simulink subsystem "Joystick_Input_To_Swerve_Drive_sub"  (R2023b)
settings: Solver=VariableStepAuto  StartTime=0.0  StopTime=10.0  RelTol=1e-3
undefined symbols (not defined in the file): Boost_Trigger_High_Speed, Boost_Trigger_Low_Speed, Steering_Abs_Deadband_Range, Steering_Mod_Drv_in, Steering_Mod_Drv_out, Steering_Mod_Str_Rel_in, Steering_Mod_Str_Rel_out, Steering_Relative_Gain, Steering_Twist_Gain, Translation_Twist_Gain
libraries: simulink x12, hdlsllib x5, Controls_Components_lib x1
settings Model: Creator=ander  LastModifiedBy=ander

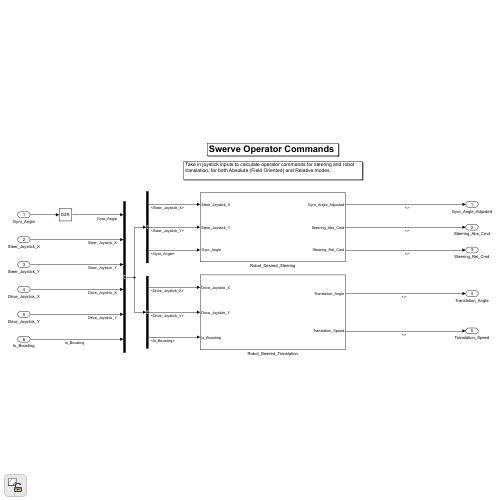
[thumbnail: Simulink's stored preview of the top-level diagram]
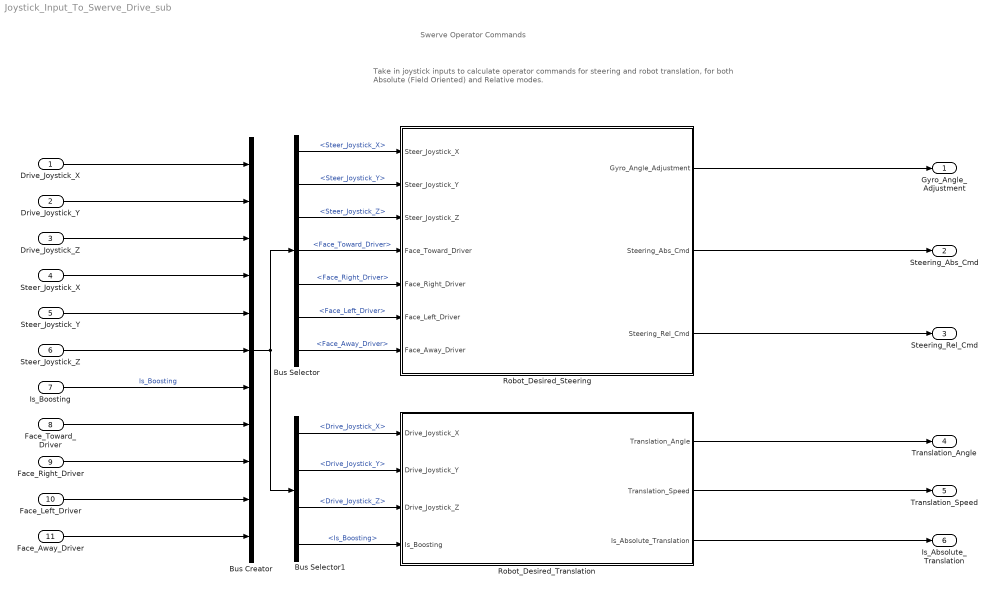
== system Joystick_Input_To_Swerve_Drive_sub ==
  note: Take in joystick inputs to calculate operator commands for steering and robot translation, for both Absolute (Field Oriented) and Relative modes.
  note: Swerve Operator Commands
  Drive_Joystick_X : Inport
  Drive_Joystick_Y : Inport  Port=2
  Drive_Joystick_Z : Inport  Port=3
  Steer_Joystick_X : Inport  Port=4
  Steer_Joystick_Y : Inport  Port=5
  Steer_Joystick_Z : Inport  Port=6
  Is_Boosting : Inport  Port=7
  Face_Toward_Driver : Inport  Port=8
  Face_Right_Driver : Inport  Port=9
  Face_Left_Driver : Inport  Port=10
  Face_Away_Driver : Inport  Port=11
  Bus Creator : BusCreator  Inputs=11
  Bus Selector : BusSelector  OutputSignals=Steer_Joystick_X,Steer_Joystick_Y,Steer_Joystick_Z,Face_Toward_Driver,Face_Right_Driver,Face_Left_Driver,Face_Away_Driver
  Bus Selector1 : BusSelector  OutputSignals=Drive_Joystick_X,Drive_Joystick_Y,Drive_Joystick_Z,Is_Boosting
  Robot_Desired_Steering : Subsystem
  Robot_Desired_Translation : Subsystem
  Gyro_Angle_Adjustment : Outport
  Steering_Abs_Cmd : Outport  Port=2
  Steering_Rel_Cmd : Outport  Port=3
  Translation_Angle : Outport  Port=4
  Translation_Speed : Outport  Port=5
  Is_Absolute_Translation : Outport  Port=6
  wires:
  Bus Selector/7 -> Robot_Desired_Steering/7(Face_Away_Driver)  "<Face_Away_Driver>"
  Bus Selector/6 -> Robot_Desired_Steering/6(Face_Left_Driver)  "<Face_Left_Driver>"
  Bus Selector/5 -> Robot_Desired_Steering/5(Face_Right_Driver)  "<Face_Right_Driver>"
  Bus Selector/3 -> Robot_Desired_Steering/3(Steer_Joystick_Z)  "<Steer_Joystick_Z>"
  Bus Selector/4 -> Robot_Desired_Steering/4(Face_Toward_Driver)  "<Face_Toward_Driver>"
  Is_Boosting/1 -> Bus Creator/7  "Is_Boosting"
  Face_Away_Driver/1 -> Bus Creator/11
  Face_Left_Driver/1 -> Bus Creator/10
  Face_Right_Driver/1 -> Bus Creator/9
  Face_Toward_Driver/1 -> Bus Creator/8
  Steer_Joystick_Z/1 -> Bus Creator/6
  Steer_Joystick_X/1 -> Bus Creator/4
  Drive_Joystick_Y/1 -> Bus Creator/2
  Steer_Joystick_Y/1 -> Bus Creator/5
  Drive_Joystick_Z/1 -> Bus Creator/3
  Drive_Joystick_X/1 -> Bus Creator/1
  Bus Selector1/1 -> Robot_Desired_Translation/1(Drive_Joystick_X)  "<Drive_Joystick_X>"
  Bus Selector1/2 -> Robot_Desired_Translation/2(Drive_Joystick_Y)  "<Drive_Joystick_Y>"
  Bus Creator/1 -> Bus Selector1/1, Bus Selector/1
  Robot_Desired_Translation/2(Translation_Speed) -> Translation_Speed/1
  Robot_Desired_Translation/1(Translation_Angle) -> Translation_Angle/1
  Bus Selector/1 -> Robot_Desired_Steering/1(Steer_Joystick_X)  "<Steer_Joystick_X>"
  Bus Selector/2 -> Robot_Desired_Steering/2(Steer_Joystick_Y)  "<Steer_Joystick_Y>"
  Robot_Desired_Steering/1(Gyro_Angle_Adjustment) -> Gyro_Angle_Adjustment/1
  Robot_Desired_Steering/2(Steering_Abs_Cmd) -> Steering_Abs_Cmd/1
  Robot_Desired_Steering/3(Steering_Rel_Cmd) -> Steering_Rel_Cmd/1
  Bus Selector1/4 -> Robot_Desired_Translation/4(Is_Boosting)  "<Is_Boosting>"
  Bus Selector1/3 -> Robot_Desired_Translation/3(Drive_Joystick_Z)  "<Drive_Joystick_Z>"
  Robot_Desired_Translation/3(Is_Absolute_Translation) -> Is_Absolute_Translation/1

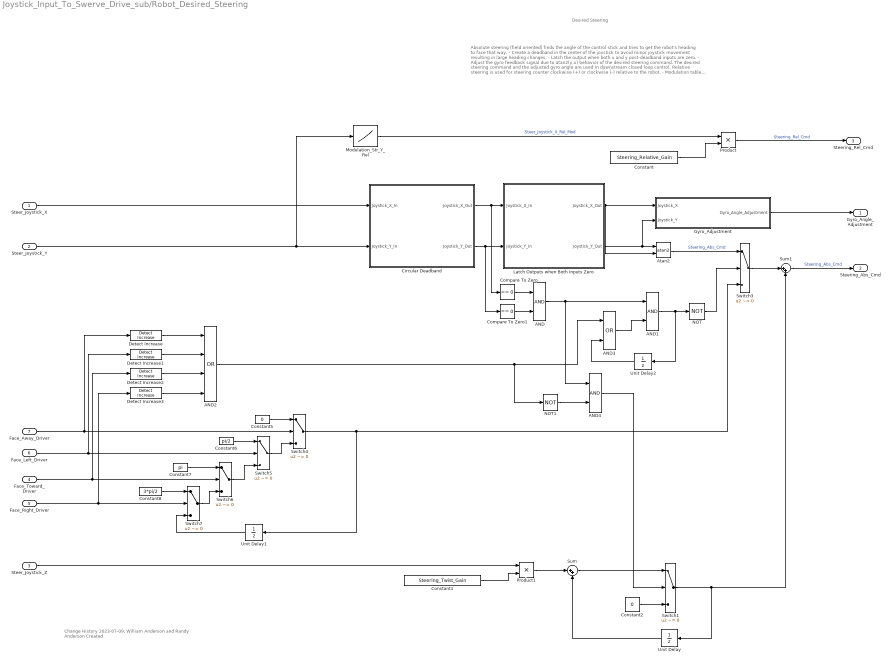
== system Joystick_Input_To_Swerve_Drive_sub/Robot_Desired_Steering ==
  note: Absolute steering (field oriented) finds the angle of the control stick and tries to get the robot's heading to face that way.
      | - Create a deadband in the center of the joystick to avoid minor joystick movement resulting in large heading changes.
      | - Latch the output when both x and y post-deadband inputs are zero.
      | - Adjust the gyro feedback signal due to atan2(y,x) behavior of the desired steering command. The desired steering command and the adjusted gyro angle are used in downstream closed loop control.
      |
      | Relative steering is used for steering counter clockwise (+) or clockwise (-) relative to the robot.
      | - Modulation table for joystick input. Only one axis of the steering joystck is used.
      | - The gain block adjusts how fast the robot will rotate.
  note: Desired Steering
  note: Change History
      | 2023-07-09, William Anderson and Randy Anderson
      | Created
  Steer_Joystick_X : Inport
  Steer_Joystick_Y : Inport  Port=2
  Steer_Joystick_Z : Inport  Port=3
  Face_Toward_Driver : Inport  Port=4
  Face_Right_Driver : Inport  Port=5
  Face_Left_Driver : Inport  Port=6
  Face_Away_Driver : Inport  Port=7
  AND : Logic  AllPortsSameDT=off  OutDataTypeStr=boolean
  AND1 : Logic  AllPortsSameDT=off  OutDataTypeStr=boolean
  AND2 : Logic  Operator=OR  Inputs=4  AllPortsSameDT=off  OutDataTypeStr=boolean
  AND3 : Logic  Operator=OR  AllPortsSameDT=off  OutDataTypeStr=boolean
  AND4 : Logic  AllPortsSameDT=off  OutDataTypeStr=boolean
  Atan2 : Trigonometry  Operator=atan2
  Circular Deadband : Subsystem
  Compare To Zero : simulink/Logic and Bit Operations/Compare To Zero  relop===  OutDataTypeStr=boolean
  Compare To Zero1 : simulink/Logic and Bit Operations/Compare To Zero  relop===  OutDataTypeStr=boolean
  Constant : Constant  Value=Steering_Relative_Gain
  Constant1 : Constant  Value=Steering_Twist_Gain
  Constant2 : Constant  Value=0
  Constant5 : Constant  Value=0
  Constant6 : Constant  Value=pi/2
  Constant7 : Constant  Value=pi
  Constant8 : Constant  Value=3*pi/2
  Detect Increase{,1..3} (4 alike) : simulink/Logic and Bit Operations/Detect Increase  vinit=0.0  OutDataTypeStr=boolean
  Gyro_Adjustment : Subsystem
  Latch Outputs when Both Inputs Zero : Subsystem
  Modulation_Str_Y_Rel : Lookup_n-D  NumberOfTableDimensions=1  BreakpointsForDimension1=Steering_Mod_Str_Rel_in  Table=Steering_Mod_Str_Rel_out  ExtrapMethod=Clip  InternalRulePriority=Speed  RndMeth=Simplest
  NOT : Logic  Operator=NOT  AllPortsSameDT=off  OutDataTypeStr=boolean
  NOT1 : Logic  Operator=NOT  AllPortsSameDT=off  OutDataTypeStr=boolean
  Product : Product
  Product1 : Product
  Sum : Sum  Inputs=|++
  Sum1 : Sum  Inputs=|++
  Switch{1,3..7} (6 alike) : Switch  Criteria=u2 ~= 0  SaturateOnIntegerOverflow=off  InputSameDT=off
  Unit Delay : UnitDelay  SampleTime=-1  HasFrameUpgradeWarning=on
  Unit Delay1 : UnitDelay  SampleTime=-1  HasFrameUpgradeWarning=on
  Unit Delay2 : UnitDelay  SampleTime=-1  HasFrameUpgradeWarning=on
  Gyro_Angle_Adjustment : Outport
  Steering_Abs_Cmd : Outport  Port=2
  Steering_Rel_Cmd : Outport  Port=3
  wires:
  NOT1/1 -> AND4/2
  AND4/1 -> Switch1/2
  Unit Delay2/1 -> AND3/2
  AND3/1 -> AND1/2
  AND1/1 -> NOT/1, Unit Delay2/1
  AND2/1 -> AND3/1, NOT1/1
  Detect Increase3/1 -> AND2/4
  Detect Increase2/1 -> AND2/3
  Detect Increase1/1 -> AND2/2
  Detect Increase/1 -> AND2/1
  Switch3/1 -> Sum1/1
  Atan2/1 -> Switch3/1  "Steering_Abs_Cmd"
  NOT/1 -> Switch3/2
  Unit Delay1/1 -> Switch7/3
  Switch4/1 -> Switch3/3, Unit Delay1/1
  Unit Delay/1 -> Sum/2
  Sum/1 -> Switch1/1
  Latch Outputs when Both Inputs Zero/1(Joystick_X_Out) -> Gyro_Adjustment/1(Joystick_X), Atan2/2
  Circular Deadband/1(Joystick_X_Out) -> Compare To Zero/1, Latch Outputs when Both Inputs Zero/1(Joystick_X_In)
  Circular Deadband/2(Joystick_Y_Out) -> Latch Outputs when Both Inputs Zero/2(Joystick_Y_In), Compare To Zero1/1
  Steer_Joystick_Y/1 -> Circular Deadband/2(Joystick_Y_In), Modulation_Str_Y_Rel/1
  Latch Outputs when Both Inputs Zero/2(Joystick_Y_Out) -> Atan2/1, Gyro_Adjustment/2(Joystick_Y)
  Gyro_Adjustment/1(Gyro_Angle_Adjustment) -> Gyro_Angle_Adjustment/1
  Sum1/1 -> Steering_Abs_Cmd/1  "Steering_Abs_Cmd"
  Constant/1 -> Product/2
  Product/1 -> Steering_Rel_Cmd/1  "Steering_Rel_Cmd"
  Steer_Joystick_X/1 -> Circular Deadband/1(Joystick_X_In)
  Modulation_Str_Y_Rel/1 -> Product/1  "Steer_Joystick_X_Rel_Mod"
  Steer_Joystick_Z/1 -> Product1/1
  Compare To Zero/1 -> AND/1
  Compare To Zero1/1 -> AND/2
  AND/1 -> AND1/1, AND4/1
  Constant2/1 -> Switch1/3
  Switch1/1 -> Unit Delay/1, Sum1/2
  Product1/1 -> Sum/1
  Constant1/1 -> Product1/2
  Constant5/1 -> Switch4/1
  Constant7/1 -> Switch6/1
  Switch6/1 -> Switch5/3
  Constant6/1 -> Switch5/1
  Constant8/1 -> Switch7/1
  Switch5/1 -> Switch4/3
  Switch7/1 -> Switch6/3
  Face_Away_Driver/1 -> Switch4/2, Detect Increase/1
  Face_Left_Driver/1 -> Switch5/2, Detect Increase1/1
  Face_Toward_Driver/1 -> Switch6/2, Detect Increase2/1
  Face_Right_Driver/1 -> Switch7/2, Detect Increase3/1

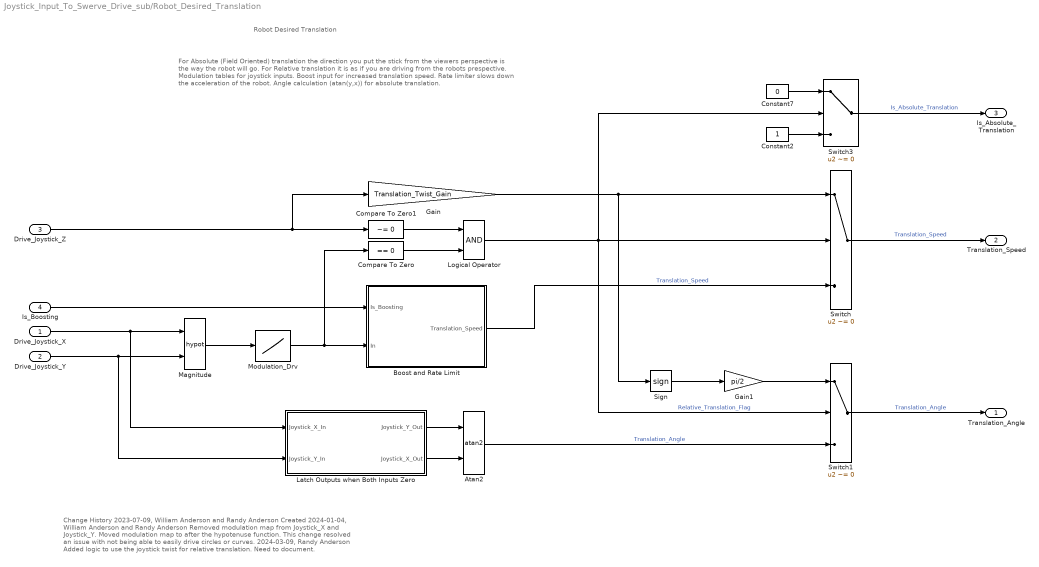
== system Joystick_Input_To_Swerve_Drive_sub/Robot_Desired_Translation ==
  note: Robot Desired Translation
  note: For Absolute (Field Oriented) translation the direction you put the stick from the viewers perspective is the way the robot will go.
      |
      | For Relative translation it is as if you are driving from the robots prespective.
      |
      | Modulation tables for joystick inputs.
      | Boost input for increased translation speed.
      | Rate limiter slows down the acceleration of the robot.
      | Angle calculation (atan(y,x)) for absolute translation.
  note: Change History
      | 2023-07-09, William Anderson and Randy Anderson
      | Created
      | 2024-01-04, William Anderson and Randy Anderson
      | Removed modulation map from Joystick_X and Joystick_Y.
      | Moved modulation map to after the hypotenuse function.
      | This change resolved an issue with not being able to easily drive circles or curves.
      | 2024-03-09, Randy Anderson
      | Added logic to use the joystick twist for relative translation. Need to document.
  Drive_Joystick_X : Inport
  Drive_Joystick_Y : Inport  Port=2
  Drive_Joystick_Z : Inport  Port=3
  Is_Boosting : Inport  Port=4
  Atan2 : Trigonometry  Operator=atan2
  Boost and Rate Limit : Subsystem
  Compare To Zero : simulink/Logic and Bit Operations/Compare To Zero  relop===  OutDataTypeStr=boolean
  Compare To Zero1 : simulink/Logic and Bit Operations/Compare To Zero  relop=~=  OutDataTypeStr=boolean
  Constant2 : Constant  OutDataTypeStr=Inherit: Inherit via back propagation
  Constant7 : Constant  Value=0  OutDataTypeStr=Inherit: Inherit via back propagation
  Gain : Gain  Gain=Translation_Twist_Gain
  Gain1 : Gain  Gain=pi/2
  Latch Outputs when Both Inputs Zero : Subsystem
  Logical Operator : Logic  AllPortsSameDT=off  OutDataTypeStr=boolean
  Magnitude : Math  Operator=hypot
  Modulation_Drv : Lookup_n-D  NumberOfTableDimensions=1  BreakpointsForDimension1=Steering_Mod_Drv_in  Table=Steering_Mod_Drv_out  ExtrapMethod=Clip  InternalRulePriority=Speed  RndMeth=Simplest
  Sign : Signum
  Switch : Switch  Criteria=u2 ~= 0  SaturateOnIntegerOverflow=off  InputSameDT=off
  Switch1 : Switch  Criteria=u2 ~= 0  SaturateOnIntegerOverflow=off  InputSameDT=off
  Switch3 : Switch  Criteria=u2 ~= 0  SaturateOnIntegerOverflow=off  InputSameDT=off
  Translation_Angle : Outport
  Translation_Speed : Outport  Port=2
  Is_Absolute_Translation : Outport  Port=3
  wires:
  Gain1/1 -> Switch1/1
  Sign/1 -> Gain1/1
  Switch3/1 -> Is_Absolute_Translation/1  "Is_Absolute_Translation"
  Constant7/1 -> Switch3/1
  Constant2/1 -> Switch3/3
  Atan2/1 -> Switch1/3  "Translation_Angle"
  Gain/1 -> Switch/1, Sign/1
  Compare To Zero/1 -> Logical Operator/2
  Compare To Zero1/1 -> Logical Operator/1
  Boost and Rate Limit/1(Translation_Speed) -> Switch/3  "Translation_Speed"
  Logical Operator/1 -> Switch3/2, Switch1/2, Switch/2  "Relative_Translation_Flag"
  Drive_Joystick_Z/1 -> Compare To Zero1/1, Gain/1
  Latch Outputs when Both Inputs Zero/1(Joystick_Y_Out) -> Atan2/1
  Latch Outputs when Both Inputs Zero/2(Joystick_X_Out) -> Atan2/2
  Is_Boosting/1 -> Boost and Rate Limit/1(Is_Boosting)
  Switch/1 -> Translation_Speed/1  "Translation_Speed"
  Switch1/1 -> Translation_Angle/1  "Translation_Angle"
  Magnitude/1 -> Modulation_Drv/1
  Drive_Joystick_X/1 -> Magnitude/1, Latch Outputs when Both Inputs Zero/1(Joystick_X_In)
  Drive_Joystick_Y/1 -> Magnitude/2, Latch Outputs when Both Inputs Zero/2(Joystick_Y_In)
  Modulation_Drv/1 -> Compare To Zero/1, Boost and Rate Limit/2(In)

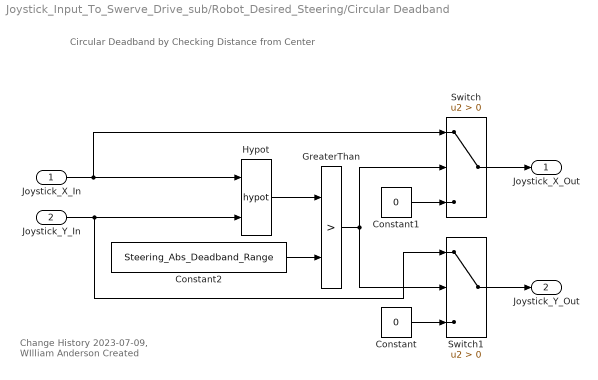
== system Joystick_Input_To_Swerve_Drive_sub/Robot_Desired_Steering/Circular Deadband ==
  note: Circular Deadband by Checking Distance from Center
  note: Change History
      | 2023-07-09, WIlliam Anderson
      | Created
  Joystick_X_In : Inport
  Joystick_Y_In : Inport  Port=2
  Constant : Constant  Value=0
  Constant1 : Constant  Value=0
  Constant2 : Constant  Value=Steering_Abs_Deadband_Range
  GreaterThan : RelationalOperator  Operator=>  OutDataTypeStr=boolean  RndMeth=Simplest  InputSameDT=off
  Hypot : Math  Operator=hypot
  Switch : Switch  Criteria=u2 > Threshold  SaturateOnIntegerOverflow=off  InputSameDT=off
  Switch1 : Switch  Criteria=u2 > Threshold  SaturateOnIntegerOverflow=off  InputSameDT=off
  Joystick_X_Out : Outport
  Joystick_Y_Out : Outport  Port=2
  wires:
  GreaterThan/1 -> Switch1/2, Switch/2
  Constant2/1 -> GreaterThan/2
  Hypot/1 -> GreaterThan/1
  Joystick_Y_In/1 -> Hypot/2, Switch1/1
  Joystick_X_In/1 -> Switch/1, Hypot/1
  Constant1/1 -> Switch/3
  Constant/1 -> Switch1/3
  Switch/1 -> Joystick_X_Out/1
  Switch1/1 -> Joystick_Y_Out/1

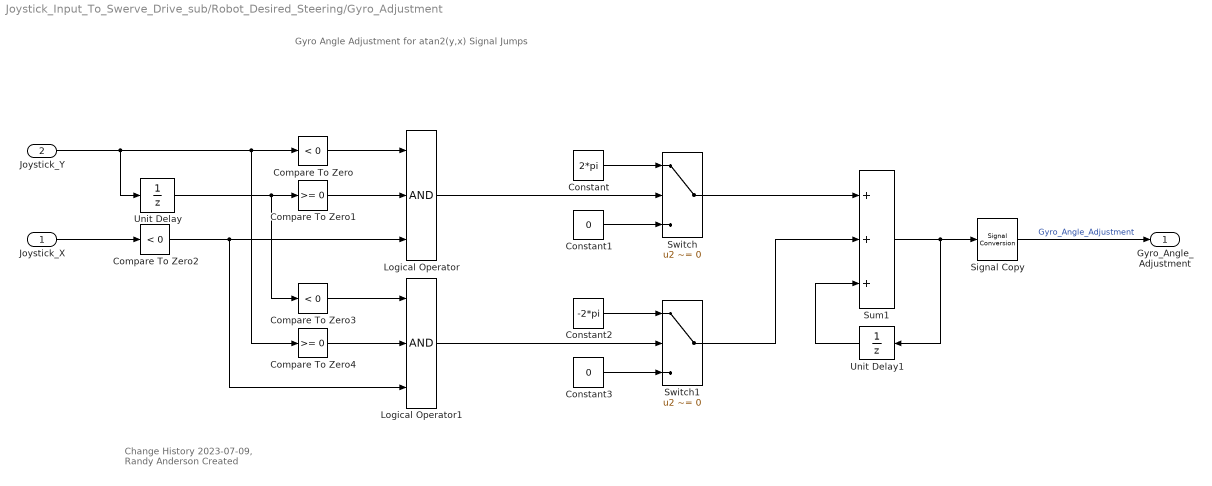
== system Joystick_Input_To_Swerve_Drive_sub/Robot_Desired_Steering/Gyro_Adjustment ==
  note: Gyro Angle Adjustment for atan2(y,x) Signal Jumps
  note: Change History
      | 2023-07-09, Randy Anderson
      | Created
  Joystick_X : Inport
  Joystick_Y : Inport  Port=2
  Compare To Zero : hdlsllib/Logic and Bit Operations/Compare To Zero  relop=<  OutDataTypeStr=boolean
  Compare To Zero1 : hdlsllib/Logic and Bit Operations/Compare To Zero  relop=>=  OutDataTypeStr=boolean
  Compare To Zero2 : hdlsllib/Logic and Bit Operations/Compare To Zero  relop=<  OutDataTypeStr=boolean
  Compare To Zero3 : hdlsllib/Logic and Bit Operations/Compare To Zero  relop=<  OutDataTypeStr=boolean
  Compare To Zero4 : hdlsllib/Logic and Bit Operations/Compare To Zero  relop=>=  OutDataTypeStr=boolean
  Constant : Constant  Value=2*pi
  Constant1 : Constant  Value=0
  Constant2 : Constant  Value=-2*pi
  Constant3 : Constant  Value=0
  Logical Operator : Logic  Inputs=3  AllPortsSameDT=off  OutDataTypeStr=boolean
  Logical Operator1 : Logic  Inputs=3  AllPortsSameDT=off  OutDataTypeStr=boolean
  Signal Copy : SignalConversion  OverrideOpt=off
  Sum1 : Sum  Inputs=3
  Switch : Switch  Criteria=u2 ~= 0  SaturateOnIntegerOverflow=off  InputSameDT=off
  Switch1 : Switch  Criteria=u2 ~= 0  SaturateOnIntegerOverflow=off  InputSameDT=off
  Unit Delay : UnitDelay  SampleTime=-1  HasFrameUpgradeWarning=on
  Unit Delay1 : UnitDelay  SampleTime=-1  HasFrameUpgradeWarning=on
  Gyro_Angle_Adjustment : Outport
  wires:
  Joystick_Y/1 -> Compare To Zero4/1, Compare To Zero/1, Unit Delay/1
  Unit Delay/1 -> Compare To Zero3/1, Compare To Zero1/1
  Compare To Zero/1 -> Logical Operator/1
  Compare To Zero1/1 -> Logical Operator/2
  Constant/1 -> Switch/1
  Constant1/1 -> Switch/3
  Logical Operator/1 -> Switch/2
  Sum1/1 -> Unit Delay1/1, Signal Copy/1
  Switch/1 -> Sum1/1
  Unit Delay1/1 -> Sum1/3
  Joystick_X/1 -> Compare To Zero2/1
  Compare To Zero2/1 -> Logical Operator1/3, Logical Operator/3
  Compare To Zero3/1 -> Logical Operator1/1
  Compare To Zero4/1 -> Logical Operator1/2
  Logical Operator1/1 -> Switch1/2
  Constant3/1 -> Switch1/3
  Constant2/1 -> Switch1/1
  Switch1/1 -> Sum1/2
  Signal Copy/1 -> Gyro_Angle_Adjustment/1  "Gyro_Angle_Adjustment"

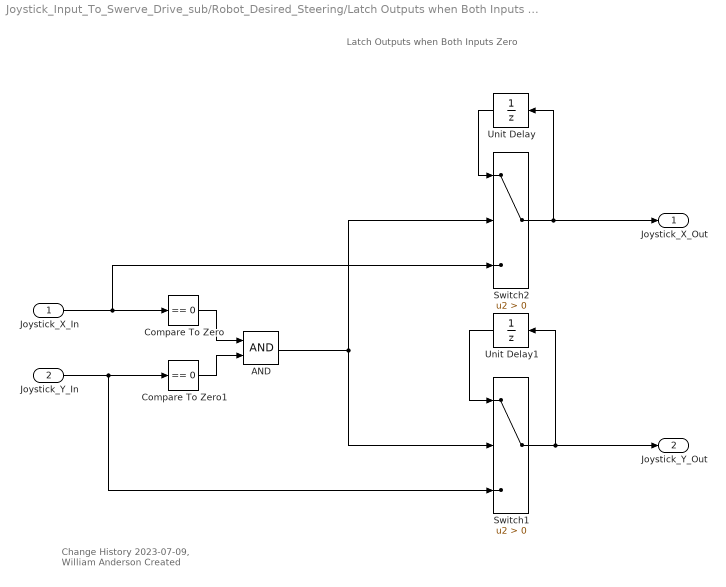
== system Joystick_Input_To_Swerve_Drive_sub/Robot_Desired_Steering/Latch Outputs when Both Inputs Zero ==
  note: Latch Outputs when Both Inputs Zero
  note: Change History
      | 2023-07-09, William Anderson
      | Created
  Joystick_X_In : Inport
  Joystick_Y_In : Inport  Port=2
  AND : Logic  AllPortsSameDT=off  OutDataTypeStr=boolean
  Compare To Zero : simulink/Logic and Bit Operations/Compare To Zero  relop===  OutDataTypeStr=boolean
  Compare To Zero1 : simulink/Logic and Bit Operations/Compare To Zero  relop===  OutDataTypeStr=boolean
  Switch1 : Switch  Criteria=u2 > Threshold  SaturateOnIntegerOverflow=off  InputSameDT=off
  Switch2 : Switch  Criteria=u2 > Threshold  SaturateOnIntegerOverflow=off  InputSameDT=off
  Unit Delay : UnitDelay  SampleTime=-1  HasFrameUpgradeWarning=on
  Unit Delay1 : UnitDelay  SampleTime=-1  HasFrameUpgradeWarning=on
  Joystick_X_Out : Outport
  Joystick_Y_Out : Outport  Port=2
  wires:
  Unit Delay1/1 -> Switch1/1
  Unit Delay/1 -> Switch2/1
  AND/1 -> Switch2/2, Switch1/2
  Compare To Zero/1 -> AND/1
  Compare To Zero1/1 -> AND/2
  Joystick_Y_In/1 -> Compare To Zero1/1, Switch1/3
  Joystick_X_In/1 -> Compare To Zero/1, Switch2/3
  Switch2/1 -> Unit Delay/1, Joystick_X_Out/1
  Switch1/1 -> Unit Delay1/1, Joystick_Y_Out/1

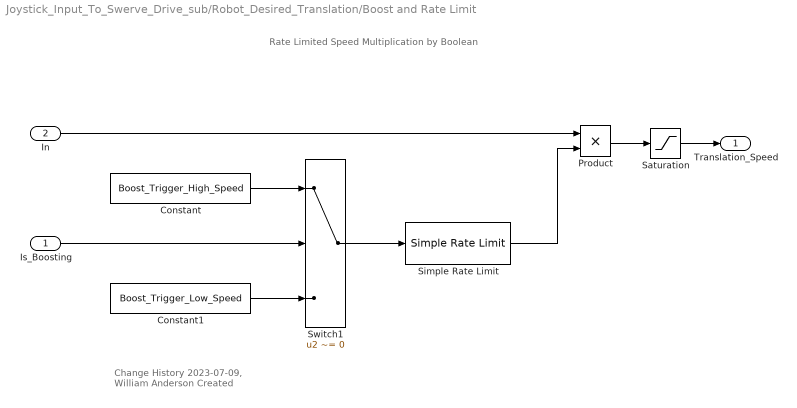
== system Joystick_Input_To_Swerve_Drive_sub/Robot_Desired_Translation/Boost and Rate Limit ==
  note: Rate Limited Speed Multiplication by Boolean
  note: Change History
      | 2023-07-09, William Anderson
      | Created
  Is_Boosting : Inport
  In : Inport  Port=2
  Constant : Constant  Value=Boost_Trigger_High_Speed
  Constant1 : Constant  Value=Boost_Trigger_Low_Speed
  Product : Product
  Saturation : Saturate  UpperLimit=Boost_Trigger_High_Speed  LowerLimit=-Boost_Trigger_High_Speed
  Simple Rate Limit : Controls_Components_lib/Simple Rate Limit  Rate_Limit_Inc=Boost_Trigger_Increasing_Limit  Rate_Limit_Dec=Boost_Trigger_Decreasing_Limit
  Switch1 : Switch  Criteria=u2 ~= 0  SaturateOnIntegerOverflow=off  InputSameDT=off
  Translation_Speed : Outport
  wires:
  Saturation/1 -> Translation_Speed/1
  Simple Rate Limit/1 -> Product/2
  Product/1 -> Saturation/1
  In/1 -> Product/1
  Switch1/1 -> Simple Rate Limit/1
  Constant1/1 -> Switch1/3
  Constant/1 -> Switch1/1
  Is_Boosting/1 -> Switch1/2

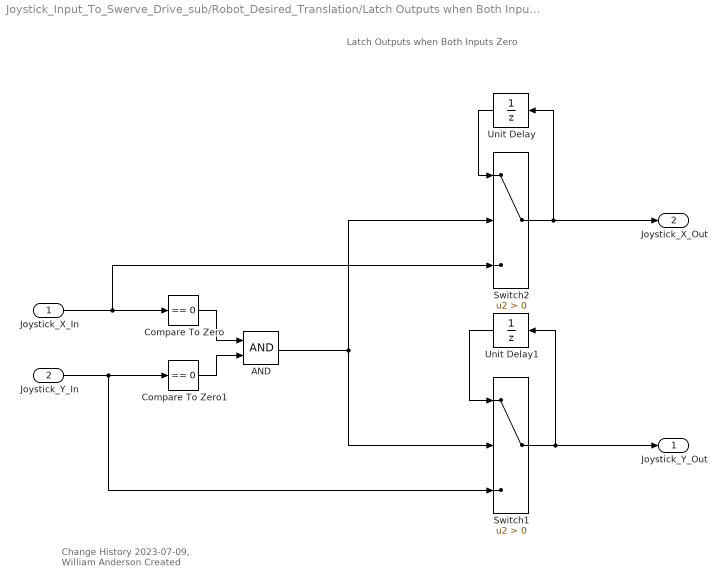
== system Joystick_Input_To_Swerve_Drive_sub/Robot_Desired_Translation/Latch Outputs when Both Inputs Zero ==
  note: Latch Outputs when Both Inputs Zero
  note: Change History
      | 2023-07-09, William Anderson
      | Created
  Joystick_X_In : Inport
  Joystick_Y_In : Inport  Port=2
  AND : Logic  AllPortsSameDT=off  OutDataTypeStr=boolean
  Compare To Zero : simulink/Logic and Bit Operations/Compare To Zero  relop===  OutDataTypeStr=boolean
  Compare To Zero1 : simulink/Logic and Bit Operations/Compare To Zero  relop===  OutDataTypeStr=boolean
  Switch1 : Switch  Criteria=u2 > Threshold  SaturateOnIntegerOverflow=off  InputSameDT=off
  Switch2 : Switch  Criteria=u2 > Threshold  SaturateOnIntegerOverflow=off  InputSameDT=off
  Unit Delay : UnitDelay  SampleTime=-1  HasFrameUpgradeWarning=on
  Unit Delay1 : UnitDelay  SampleTime=-1  HasFrameUpgradeWarning=on
  Joystick_Y_Out : Outport
  Joystick_X_Out : Outport  Port=2
  wires:
  Unit Delay1/1 -> Switch1/1
  Unit Delay/1 -> Switch2/1
  AND/1 -> Switch2/2, Switch1/2
  Compare To Zero/1 -> AND/1
  Compare To Zero1/1 -> AND/2
  Joystick_Y_In/1 -> Compare To Zero1/1, Switch1/3
  Joystick_X_In/1 -> Compare To Zero/1, Switch2/3
  Switch2/1 -> Unit Delay/1, Joystick_X_Out/1
  Switch1/1 -> Unit Delay1/1, Joystick_Y_Out/1
